simulink model "PID_ControllerJan18"  (R2023b)
settings: Solver=VariableStepAuto  StartTime=0.0  StopTime=100  RelTol=1e-3
libraries: slpidlib x2
settings Model: Creator=abbas  LastModifiedBy=ericliang
settings OptimizationCC: ReuseModelBlockBuffer=off

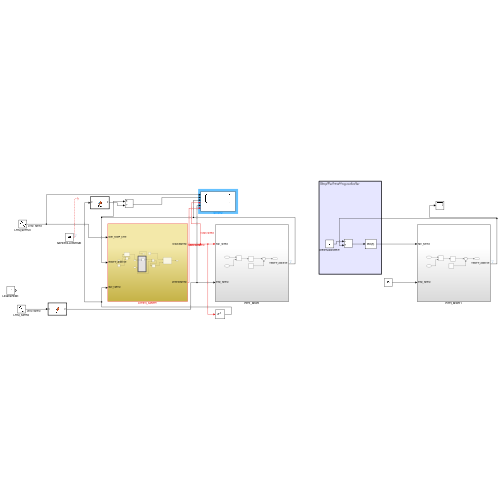
[thumbnail: Simulink's stored preview of the top-level diagram]
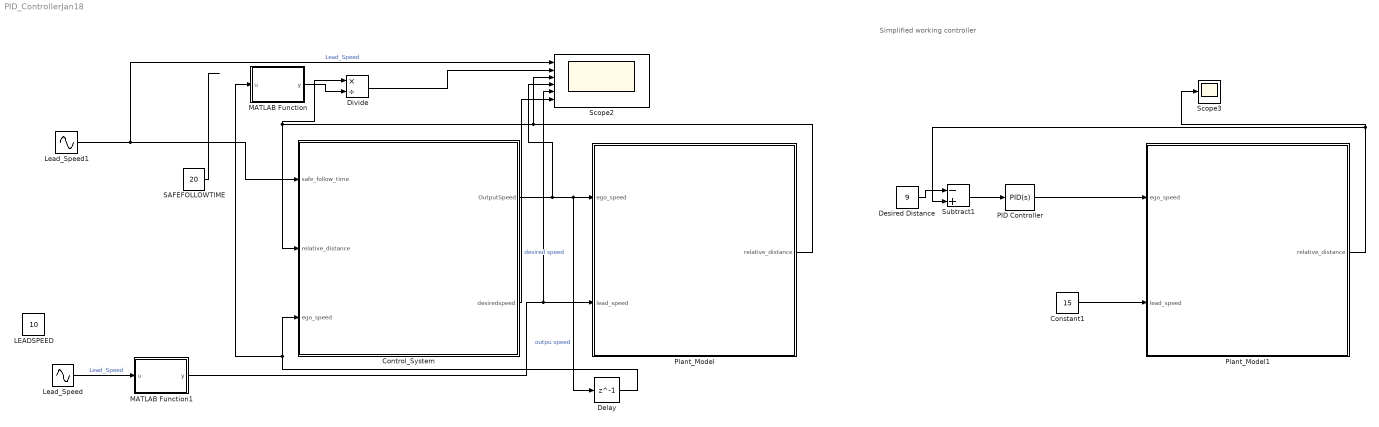
== system PID_ControllerJan18 ==
  note: Simplified working controller
  Constant1 : Constant  Value=15
  Control_System : Subsystem
  Delay : Delay  DelayLength=1  InitialCondition=0  SampleTime=0.1
  Desired Distance : Constant  Value=9
  Divide : Product  Inputs=*/
  LEADSPEED : Constant  Value=10
  Lead_Speed : Sin  Amplitude=40  Bias=10  Frequency=.25  SampleTime=0
  Lead_Speed1 : Sin  Amplitude=0  Bias=5  Frequency=0.1  SampleTime=0
  MATLAB Function : MATLAB Function  TreatAsAtomicUnit=on
  MATLAB Function1 : MATLAB Function  TreatAsAtomicUnit=on
  PID Controller : slpidlib/PID Controller  Controller=PID  Form=Parallel  TimeDomain=Continuous-time  UseExternalTs=off  SampleTime=-1  IntegratorMethod=Forward Euler  FilterMethod=Forward Euler  ControllerParametersSource=internal  P=1  I=1  UseKiTs=off  D=0  N=100  UseFilter=on  TunerSelectOption=Transfer Function Based (PID Tuner App)  InitialConditionSource=internal  InitialConditionForIntegrator=0  InitialConditionForFilter=0  DifferentiatorICPrevScaledInput=0  ExternalReset=none  TrackingMode=off  Kt=1  LimitOutput=off  SatLimitsSource=internal  UpperSaturationLimit=inf  LowerSaturationLimit=-inf  LinearizeAsGain=on  AntiWindupMode=none  Kb=1  LimitIntegrator=off  UpperIntegratorSaturationLimit=inf  LowerIntegratorSaturationLimit=-inf  POutMin=[]  POutMax=[]  IOutMin=[]  IOutMax=[]  DOutMin=[]  DOutMax=[]  NOutMin=[]  NOutMax=[]  SumOutMin=[]  SumOutMax=[]  SaturationOutMin=[]  SaturationOutMax=[]  PParamMin=[]  PParamMax=[]  IParamMin=[]  IParamMax=[]  DParamMin=[]  DParamMax=[]  NParamMin=[]  NParamMax=[]  KbParamMin=[]  KbParamMax=[]  KtParamMin=[]  KtParamMax=[]  KbOutMin=[]  KbOutMax=[]  KtOutMin=[]  KtOutMax=[]  IntegratorOutMin=[]  IntegratorOutMax=[]  FilterOutMin=[]  FilterOutMax=[]  SumI1OutMin=[]  SumI1OutMax=[]  SumI2OutMin=[]  SumI2OutMax=[]  SumI3OutMin=[]  SumI3OutMax=[]  SumI4OutMin=[]  SumI4OutMax=[]  SumDOutMin=[]  SumDOutMax=[]  DifferentiatorOutMin=[]  DifferentiatorOutMax=[]  FilterDiffOutCoefMin=[]  FilterDiffOutCoefMax=[]  ReciprocalOutMin=[]  ReciprocalOutMax=[]  SumDenOutMin=[]  SumDenOutMax=[]  SumNumOutMin=[]  SumNumOutMax=[]  DivideOutMin=[]  DivideOutMax=[]  UdiffTsProdOutMin=[]  UdiffTsProdOutMax=[]  NTsProdOutMin=[]  NTsProdOutMax=[]  UintegralTsProdOutMin=[]  UintegralTsProdOutMax=[]  UngainTsProdOutMin=[]  UngainTsProdOutMax=[]  ClampingZeroOutDataTypeStr=Inherit: Inherit via back propagation  ClampingZeroOutMin=[]  ClampingZeroOutMax=[]  FilterDenConstantOutDataTypeStr=Inherit: Inherit via back propagation  FilterDenConstantOutMin=[]  FilterDenConstantOutMax=[]  PCopyOutDataTypeStr=Inherit: Inherit via back propagation  PCopyOutMin=[]  PCopyOutMax=[]  NCopyOutDataTypeStr=Inherit: Inherit via back propagation  NCopyOutMin=[]  NCopyOutMax=[]  IntegratorContinuousStateAttributes=''  IntegratorStateMustResolveToSignalObject=off  IntegratorRTWStateStorageClass=Auto  FilterContinuousStateAttributes=''  FilterStateMustResolveToSignalObject=off  FilterRTWStateStorageClass=Auto  ParallelPVariant=InternalParameters  IdealPVariant=Disabled  IVariant=InternalParameters  DVariant=InternalParameters  IntegratorVariant=Continuous  SatVariant=Disabled  AWVariant=Passthrough  PCopyVariant=Disabled  TRVariant=Disabled  FdbkBlocksVariant=Forward  IdealPFdbkVariant=Disabled  SatFdbkVariant=Disabled  DerivativeFilterVariant=ContFilter  NVariant=InternalParameters  NCopyVariant=Disabled  FilterICVariant=InternalICsFilter  IntegratorICVariant=InternalICs  ExternalResetVariant=Disabled  TRSumVariant=Passthrough  SumFdbkVariant=Disabled  SumVariant=Sum_PID  TsampFilterVariant=InternalTs  TsampNgainVariant=Passthrough  TsampIntegralVariant=Disabled_SignalSpec  ExternalSaturationOutDataTypeStr=Inherit: Same as second input
  Plant_Model : Subsystem
  Plant_Model1 : Subsystem
  SAFEFOLLOWTIME : Constant  Value=20
  Scope2 : Scope  NumInputPorts=6
  Scope3 : Scope
  Subtract1 : Sum  Inputs=-+
  wires:
  Plant_Model/1(relative_distance) -> Scope2/3, Control_System/2(relative_distance), Divide/1
  SAFEFOLLOWTIME/1 -> ?
  Control_System/1(OutputSpeed) -> Scope2/4, Delay/1, Plant_Model/1(ego_speed)  "outpu speed"
  Constant1/1 -> Plant_Model1/2(lead_speed)
  Plant_Model1/1(relative_distance) -> Subtract1/2, Scope3/1
  Desired Distance/1 -> Subtract1/1
  Subtract1/1 -> PID Controller/1
  PID Controller/1 -> Plant_Model1/1(ego_speed)
  Delay/1 -> MATLAB Function/1(u), Control_System/3(ego_speed)
  Lead_Speed/1 -> MATLAB Function1/1(u)  "Lead_Speed"
  Lead_Speed1/1 -> Scope2/1, Control_System/1(safe_follow_time)  "Lead_Speed"
  MATLAB Function/1(y) -> Divide/2
  Divide/1 -> Scope2/2
  MATLAB Function1/1(y) -> Plant_Model/2(lead_speed), Scope2/5
  Control_System/2(desiredspeed) -> Scope2/6  "desired speed"

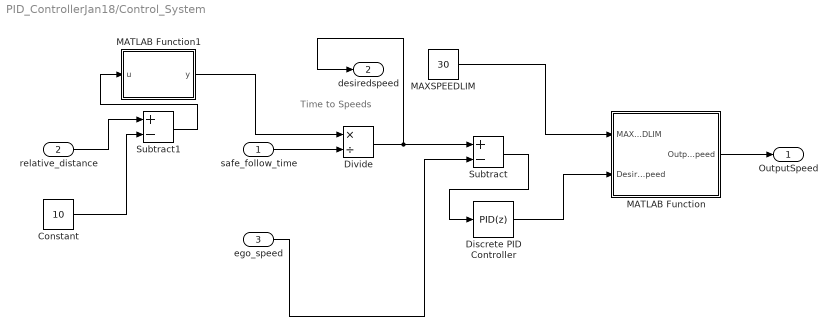
== system PID_ControllerJan18/Control_System ==
  note: Time to Speeds
  safe_follow_time : Inport
  relative_distance : Inport  Port=2
  ego_speed : Inport  Port=3
  Constant : Constant  Value=10
  Discrete PID Controller : slpidlib/PID Controller  Controller=PID  Form=Parallel  TimeDomain=Discrete-time  UseExternalTs=off  SampleTime=-1  IntegratorMethod=Forward Euler  FilterMethod=Forward Euler  ControllerParametersSource=internal  P=1.2  I=1  UseKiTs=on  D=0  N=100  UseFilter=on  TunerSelectOption=Transfer Function Based (PID Tuner App)  InitialConditionSource=internal  InitialConditionForIntegrator=0  InitialConditionForFilter=0  DifferentiatorICPrevScaledInput=0  ExternalReset=none  TrackingMode=off  Kt=1  LimitOutput=off  SatLimitsSource=internal  UpperSaturationLimit=inf  LowerSaturationLimit=-inf  LinearizeAsGain=off  AntiWindupMode=none  Kb=1  LimitIntegrator=off  UpperIntegratorSaturationLimit=inf  LowerIntegratorSaturationLimit=-inf  POutMin=[]  POutMax=[]  IOutMin=[]  IOutMax=[]  DOutMin=[]  DOutMax=[]  NOutMin=[]  NOutMax=[]  SumOutMin=[]  SumOutMax=[]  SaturationOutMin=[]  SaturationOutMax=[]  PParamMin=[]  PParamMax=[]  IParamMin=[]  IParamMax=[]  DParamMin=[]  DParamMax=[]  NParamMin=[]  NParamMax=[]  KbParamMin=[]  KbParamMax=[]  KtParamMin=[]  KtParamMax=[]  KbOutMin=[]  KbOutMax=[]  KtOutMin=[]  KtOutMax=[]  IntegratorOutMin=[]  IntegratorOutMax=[]  FilterOutMin=[]  FilterOutMax=[]  SumI1OutMin=[]  SumI1OutMax=[]  SumI2OutMin=[]  SumI2OutMax=[]  SumI3OutMin=[]  SumI3OutMax=[]  SumI4OutMin=[]  SumI4OutMax=[]  SumDOutMin=[]  SumDOutMax=[]  DifferentiatorOutMin=[]  DifferentiatorOutMax=[]  FilterDiffOutCoefMin=[]  FilterDiffOutCoefMax=[]  ReciprocalOutMin=[]  ReciprocalOutMax=[]  SumDenOutMin=[]  SumDenOutMax=[]  SumNumOutMin=[]  SumNumOutMax=[]  DivideOutMin=[]  DivideOutMax=[]  UdiffTsProdOutMin=[]  UdiffTsProdOutMax=[]  NTsProdOutMin=[]  NTsProdOutMax=[]  UintegralTsProdOutMin=[]  UintegralTsProdOutMax=[]  UngainTsProdOutMin=[]  UngainTsProdOutMax=[]  ClampingZeroOutDataTypeStr=Inherit: Inherit via back propagation  ClampingZeroOutMin=[]  ClampingZeroOutMax=[]  FilterDenConstantOutDataTypeStr=Inherit: Inherit via back propagation  FilterDenConstantOutMin=[]  FilterDenConstantOutMax=[]  PCopyOutDataTypeStr=Inherit: Inherit via back propagation  PCopyOutMin=[]  PCopyOutMax=[]  NCopyOutDataTypeStr=Inherit: Inherit via back propagation  NCopyOutMin=[]  NCopyOutMax=[]  IntegratorContinuousStateAttributes=''  IntegratorStateMustResolveToSignalObject=off  IntegratorRTWStateStorageClass=Auto  FilterContinuousStateAttributes=''  FilterStateMustResolveToSignalObject=off  FilterRTWStateStorageClass=Auto  ParallelPVariant=InternalParameters  IdealPVariant=Disabled  IVariant=InternalParameters  DVariant=InternalParameters  IntegratorVariant=Discrete  SatVariant=Disabled  AWVariant=Passthrough  PCopyVariant=Disabled  TRVariant=Disabled  FdbkBlocksVariant=Forward  IdealPFdbkVariant=Disabled  SatFdbkVariant=Disabled  DerivativeFilterVariant=ForwardEulerFilter  NVariant=InternalParameters  NCopyVariant=Disabled  FilterICVariant=InternalICsFilter  IntegratorICVariant=InternalICs  ExternalResetVariant=Disabled  TRSumVariant=Passthrough  SumFdbkVariant=Disabled  SumVariant=Sum_PID  TsampFilterVariant=InternalTs  TsampNgainVariant=Passthrough  TsampIntegralVariant=Disabled_SignalSpec  ExternalSaturationOutDataTypeStr=Inherit: Same as second input
      settings: LibrarySourceBlock=simulink/Discrete/Discrete PID Controller
  Divide : Product  Inputs=*/
  MATLAB Function : MATLAB Function  TreatAsAtomicUnit=on
  MATLAB Function1 : MATLAB Function  TreatAsAtomicUnit=on
  MAXSPEEDLIM : Constant  Value=30
  Subtract : Sum  Inputs=+-
  Subtract1 : Sum  Inputs=+-
  OutputSpeed : Outport
  desiredspeed : Outport  Port=2
  wires:
  safe_follow_time/1 -> Divide/2
  MAXSPEEDLIM/1 -> MATLAB Function/1(MAXSPEEDLIM)
  MATLAB Function/1(Output_Speed) -> OutputSpeed/1
  Divide/1 -> desiredspeed/1, Subtract/1
  ego_speed/1 -> Subtract/2
  Discrete PID Controller/1 -> MATLAB Function/2(DesiredSpeed)
  Subtract/1 -> Discrete PID Controller/1
  relative_distance/1 -> Subtract1/1
  MATLAB Function1/1(y) -> Divide/1
  Constant/1 -> Subtract1/2
  Subtract1/1 -> MATLAB Function1/1(u)

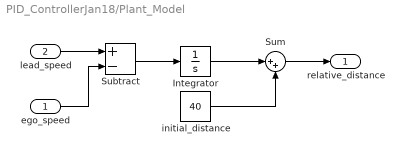
== system PID_ControllerJan18/Plant_Model ==
  ego_speed : Inport
  lead_speed : Inport  Port=2
  Integrator : Integrator
  Subtract : Sum  Inputs=+-
  Sum : Sum  Inputs=|++
  initial_distance : Constant  Value=40
  relative_distance : Outport
  wires:
  lead_speed/1 -> Subtract/1
  Subtract/1 -> Integrator/1
  ego_speed/1 -> Subtract/2
  Integrator/1 -> Sum/1
  initial_distance/1 -> Sum/2
  Sum/1 -> relative_distance/1

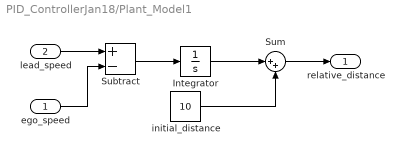
== system PID_ControllerJan18/Plant_Model1 ==
  ego_speed : Inport
  lead_speed : Inport  Port=2
  Integrator : Integrator
  Subtract : Sum  Inputs=+-
  Sum : Sum  Inputs=|++
  initial_distance : Constant  Value=10
  relative_distance : Outport
  wires:
  lead_speed/1 -> Subtract/1
  Subtract/1 -> Integrator/1
  ego_speed/1 -> Subtract/2
  Integrator/1 -> Sum/1
  initial_distance/1 -> Sum/2
  Sum/1 -> relative_distance/1

== matlab function PID_ControllerJan18/Control_System/MATLAB Function ==
  data: MAXSPEEDLIM input; Output_Speed output; DesiredSpeed input
function Output_Speed = fcn(MAXSPEEDLIM, DesiredSpeed)

if DesiredSpeed >= MAXSPEEDLIM
    Output_Speed = MAXSPEEDLIM;
elseif DesiredSpeed < 0
    Output_Speed = 0;
else 
    Output_Speed = DesiredSpeed;

end

== matlab function PID_ControllerJan18/MATLAB Function1 ==
  data: u input; y output
function y = fcn(u)

if u < 0
    y = 0;
else
    y = u;
end

== matlab function PID_ControllerJan18/Control_System/MATLAB Function1 ==
  data: u input; y output
function y = fcn(u)
%#codegen

if u < 0
    y = 0;
else
    y = u;
end

== matlab function PID_ControllerJan18/MATLAB Function ==
  data: u input; y output
function y = fcn(u)

if u == 0
    y = 1000;
else 
    y = u;
end
